simulink model "Lab2_part2"  (R2023a)
settings: Solver=VariableStepAuto  StartTime=0.0  StopTime=10.0  RelTol=1e-3
settings Model: Creator=huihany2  LastModifiedBy=huihany2

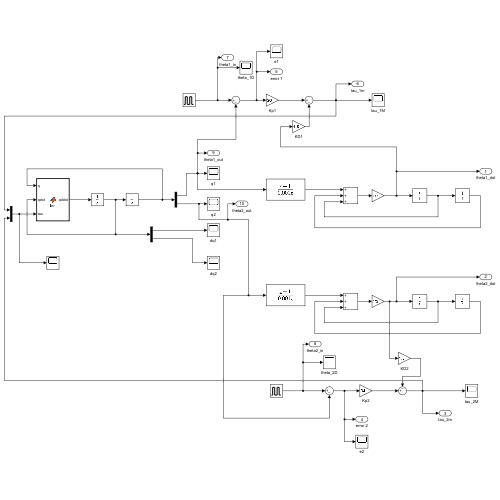
[thumbnail: Simulink's stored preview of the top-level diagram]
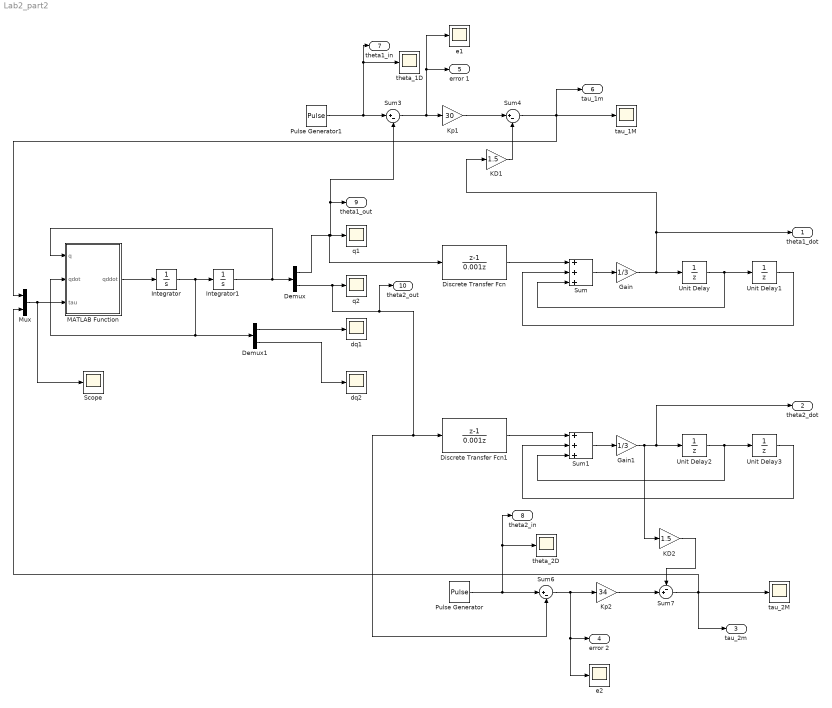
== system Lab2_part2 ==
  Demux : Demux  Outputs=2
  Demux1 : Demux  Outputs=2
  Discrete Transfer Fcn : DiscreteTransferFcn  Numerator=[1 -1]  Denominator=[0.001 0]
  Discrete Transfer Fcn1 : DiscreteTransferFcn  Numerator=[1 -1]  Denominator=[0.001 0]
  Gain : Gain  Gain=1/3
  Gain1 : Gain  Gain=1/3
  Integrator : Integrator  InitialCondition=[0;0]
  Integrator1 : Integrator  InitialCondition=[pi;pi/2]
  KD1 : Gain  Gain=1.5
  KD2 : Gain  Gain=1.5
  Kp1 : Gain  Gain=30
  Kp2 : Gain  Gain=34
  MATLAB Function : MATLAB Function  TreatAsAtomicUnit=on
  Mux : Mux  Inputs=2
  Pulse Generator : DiscretePulseGenerator  PulseType=Time based  Amplitude=pi/6  PulseWidth=50
  Pulse Generator1 : DiscretePulseGenerator  PulseType=Time based  Amplitude=pi/6  PulseWidth=50
  Scope : Scope
  Sum : Sum  Inputs=+++
  Sum1 : Sum  Inputs=+++
  Sum3 : Sum  Inputs=|+-
  Sum4 : Sum  Inputs=|+-
  Sum6 : Sum  Inputs=|+-
  Sum7 : Sum  Inputs=-+|
  Unit Delay{,1..3} (4 alike) : UnitDelay  SampleTime=0.001  HasFrameUpgradeWarning=on
  dq1 : Scope
  dq2 : Scope
  e1 : Scope
  e2 : Scope
  q1 : Scope
  q2 : Scope
  tau_1M : Scope
  tau_2M : Scope
  theta_1D : Scope
  theta_2D : Scope
  theta1_dot : Outport
  theta2_dot : Outport  Port=2
  tau_2m : Outport  Port=3
  error 2 : Outport  Port=4
  error 1 : Outport  Port=5
  tau_1m : Outport  Port=6
  theta1_in : Outport  Port=7
  theta2_in : Outport  Port=8
  theta1_out : Outport  Port=9
  theta2_out : Outport  Port=10
  wires:
  Integrator/1 -> Demux1/1, MATLAB Function/2(qdot), Integrator1/1
  Demux/1 -> theta1_out/1, Sum3/2, q1/1, Discrete Transfer Fcn/1
  Demux/2 -> theta2_out/1, Discrete Transfer Fcn1/1, Sum6/2, q2/1
  Demux1/1 -> dq1/1
  Demux1/2 -> dq2/1
  MATLAB Function/1(qddot) -> Integrator/1
  Sum4/1 -> tau_1m/1, Mux/1, tau_1M/1
  Unit Delay/1 -> Unit Delay1/1, Sum/3
  Gain/1 -> Unit Delay/1, KD1/1, theta1_dot/1
  Sum/1 -> Gain/1
  Unit Delay1/1 -> Sum/2
  Discrete Transfer Fcn/1 -> Sum/1
  Integrator1/1 -> MATLAB Function/1(q), Demux/1
  Unit Delay2/1 -> Unit Delay3/1, Sum1/3
  Discrete Transfer Fcn1/1 -> Sum1/1
  Gain1/1 -> KD2/1, theta2_dot/1, Unit Delay2/1
  Unit Delay3/1 -> Sum1/2
  Sum1/1 -> Gain1/1
  Sum3/1 -> e1/1, error 1/1, Kp1/1
  Kp1/1 -> Sum4/1
  KD1/1 -> Sum4/2
  Sum7/1 -> tau_2m/1, Mux/2, tau_2M/1
  Kp2/1 -> Sum7/2
  KD2/1 -> Sum7/1
  Pulse Generator/1 -> theta2_in/1, theta_2D/1, Sum6/1
  Mux/1 -> Scope/1, MATLAB Function/3(tau)
  Sum6/1 -> e2/1, error 2/1, Kp2/1
  Pulse Generator1/1 -> theta1_in/1, theta_1D/1, Sum3/1

== matlab function Lab2_part2/MATLAB Function ==
  data: q input; qddot output; qdot input; tau input
function qddot = fcn(q, qdot, tau)
p1 = 0.03;
p2 = 0.0128;
p3 = 0.0076;
p4 = 0.0752;
p5 = 0.0298;

tau1 = [tau(1);
        tau(2)];
g = 9.81;

D = [p1                 -p3*sin(q(2)-q(1));
    -p3*sin(q(2)-q(1))  p2];
C = [0                          -p3*cos(q(2)-q(1))*qdot(2);
    p3*cos(q(2)-q(1))*qdot(1)   0];

G = [-p4*g*sin(q(1));
    -p5*g*cos(q(2))];

qddot = D\tau1-(D\C)*qdot-D\G;
